simulink model "KillerWhaleModelPneumaticControl"  (R2020b)
settings: Solver=ode15s  StartTime=0.0  StopTime=10  MaxStep=0.01  RelTol=1e-3
model workspace: external: MATLAB File KillerWhaleParams.m (data not in the file)
undefined symbols (not defined in the file or in its folder): frontParams, rearParams, standParams, X, Y, Z
libraries: sm_lib x4301, nesl_utility x6
(part 5 of 66)

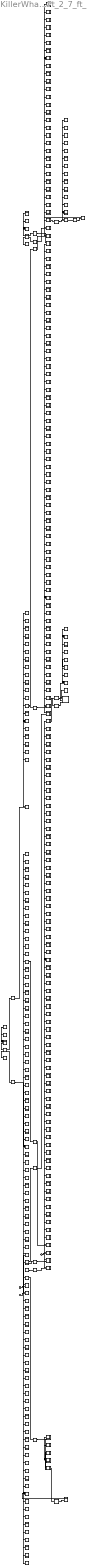
== system KillerWhaleModelPneumaticControl/RearLinkage/Tail_Linkage_Pt_2_7_ft_1 ==
  Bracket_10_RIGID : Subsystem
  Bracket_11_RIGID : Subsystem
  Bracket_12_RIGID : Subsystem
  Bracket_1_RIGID : Subsystem
  Bracket_2_RIGID : Subsystem
  Bracket_3_RIGID : Subsystem
  Bracket_4_RIGID : Subsystem
  Bracket_5_RIGID : Subsystem
  Bracket_6_RIGID : Subsystem
  Bracket_7_RIGID : Subsystem
  Bracket_8_RIGID : Subsystem
  Bracket_9_RIGID : Subsystem
  Cylindrical7 : sm_lib/Joints/Cylindrical Joint  JointMode=Normal  SenseConstraintForce=off  SenseConstraintForceX=off  SenseConstraintForceY=off  SenseConstraintForceZ=off  SenseConstraintTorque=off  SenseConstraintTorqueX=off  SenseConstraintTorqueY=off  SenseConstraintTorqueZ=off  SenseTotalForce=off  SenseTotalForceX=off  SenseTotalForceY=off  SenseTotalForceZ=off  SenseTotalTorque=off  SenseTotalTorqueX=off  SenseTotalTorqueY=off  SenseTotalTorqueZ=off  CompositeWrenchDir=FollowerOnBase  CompositeWrenchFrame=BaseFrame  PzEquilibriumPosition=0  PzEquilibriumPositionUnits=m  PzSpringStiffness=0  PzSpringStiffnessUnits=N/m  PzDampingCoefficient=0  PzDampingCoefficientUnits=N/(m/s)  PzTorqueActuationMode=NoTorque  PzMotionActuationMode=ComputedMotion  PzSensePosition=off  PzSenseVelocity=off  PzSenseAcceleration=off  PzSenseTorqueForce=off  PzSenseLowerLimitTorqueForce=off  PzSenseUpperLimitTorqueForce=off  PzLowerLimitSpecify=off  PzLowerLimitBound=-1  PzLowerLimitBoundUnits=m  PzLowerLimitStiffness=1e6  PzLowerLimitStiffnessUnits=N/m  PzLowerLimitDamping=1e3  PzLowerLimitDampingUnits=N/(m/s)  PzLowerLimitTransitionRegionWidth=1e-4  PzLowerLimitTransitionRegionWidthUnits=m  PzUpperLimitSpecify=off  PzUpperLimitBound=1  PzUpperLimitBoundUnits=m  PzUpperLimitStiffness=1e6  PzUpperLimitStiffnessUnits=N/m  PzUpperLimitDamping=1e3  PzUpperLimitDampingUnits=N/(m/s)  PzUpperLimitTransitionRegionWidth=1e-4  PzUpperLimitTransitionRegionWidthUnits=m  PzPositionTargetSpecify=off  PzPositionTargetPriority=High  PzPositionTargetValue=0  PzPositionTargetValueUnits=m  PzVelocityTargetSpecify=off  PzVelocityTargetPriority=High  PzVelocityTargetValue=0  PzVelocityTargetValueUnits=m/s  RzEquilibriumPosition=0  RzEquilibriumPositionUnits=deg  RzSpringStiffness=0  RzSpringStiffnessUnits=N*m/deg  RzDampingCoefficient=0  RzDampingCoefficientUnits=N*m/(deg/s)  RzTorqueActuationMode=NoTorque  RzMotionActuationMode=ComputedMotion  RzSensePosition=off  RzSenseVelocity=off  RzSenseAcceleration=off  RzSenseTorqueForce=off  RzSenseLowerLimitTorqueForce=off  RzSenseUpperLimitTorqueForce=off  RzLowerLimitSpecify=off  RzLowerLimitBound=-90  RzLowerLimitBoundUnits=deg  RzLowerLimitStiffness=1e4  RzLowerLimitStiffnessUnits=N*m/deg  RzLowerLimitDamping=10  RzLowerLimitDampingUnits=N*m/(deg/s)  RzLowerLimitTransitionRegionWidth=0.1  RzLowerLimitTransitionRegionWidthUnits=deg  RzUpperLimitSpecify=off  RzUpperLimitBound=90  RzUpperLimitBoundUnits=deg  RzUpperLimitStiffness=1e4  RzUpperLimitStiffnessUnits=N*m/deg  RzUpperLimitDamping=10  RzUpperLimitDampingUnits=N*m/(deg/s)  RzUpperLimitTransitionRegionWidth=0.1  RzUpperLimitTransitionRegionWidthUnits=deg  RzPositionTargetSpecify=off  RzPositionTargetPriority=High  RzPositionTargetValue=0  RzPositionTargetValueUnits=deg  RzVelocityTargetSpecify=off  RzVelocityTargetPriority=High  RzVelocityTargetValue=0  RzVelocityTargetValueUnits=deg/s
  Cylindrical8 : sm_lib/Joints/Cylindrical Joint  JointMode=Normal  SenseConstraintForce=off  SenseConstraintForceX=off  SenseConstraintForceY=off  SenseConstraintForceZ=off  SenseConstraintTorque=off  SenseConstraintTorqueX=off  SenseConstraintTorqueY=off  SenseConstraintTorqueZ=off  SenseTotalForce=off  SenseTotalForceX=off  SenseTotalForceY=off  SenseTotalForceZ=off  SenseTotalTorque=off  SenseTotalTorqueX=off  SenseTotalTorqueY=off  SenseTotalTorqueZ=off  CompositeWrenchDir=FollowerOnBase  CompositeWrenchFrame=BaseFrame  PzEquilibriumPosition=0  PzEquilibriumPositionUnits=m  PzSpringStiffness=0  PzSpringStiffnessUnits=N/m  PzDampingCoefficient=0  PzDampingCoefficientUnits=N/(m/s)  PzTorqueActuationMode=NoTorque  PzMotionActuationMode=ComputedMotion  PzSensePosition=off  PzSenseVelocity=off  PzSenseAcceleration=off  PzSenseTorqueForce=off  PzSenseLowerLimitTorqueForce=off  PzSenseUpperLimitTorqueForce=off  PzLowerLimitSpecify=off  PzLowerLimitBound=-1  PzLowerLimitBoundUnits=m  PzLowerLimitStiffness=1e6  PzLowerLimitStiffnessUnits=N/m  PzLowerLimitDamping=1e3  PzLowerLimitDampingUnits=N/(m/s)  PzLowerLimitTransitionRegionWidth=1e-4  PzLowerLimitTransitionRegionWidthUnits=m  PzUpperLimitSpecify=off  PzUpperLimitBound=1  PzUpperLimitBoundUnits=m  PzUpperLimitStiffness=1e6  PzUpperLimitStiffnessUnits=N/m  PzUpperLimitDamping=1e3  PzUpperLimitDampingUnits=N/(m/s)  PzUpperLimitTransitionRegionWidth=1e-4  PzUpperLimitTransitionRegionWidthUnits=m  PzPositionTargetSpecify=off  PzPositionTargetPriority=High  PzPositionTargetValue=0  PzPositionTargetValueUnits=m  PzVelocityTargetSpecify=off  PzVelocityTargetPriority=High  PzVelocityTargetValue=0  PzVelocityTargetValueUnits=m/s  RzEquilibriumPosition=0  RzEquilibriumPositionUnits=deg  RzSpringStiffness=0  RzSpringStiffnessUnits=N*m/deg  RzDampingCoefficient=0  RzDampingCoefficientUnits=N*m/(deg/s)  RzTorqueActuationMode=NoTorque  RzMotionActuationMode=ComputedMotion  RzSensePosition=off  RzSenseVelocity=off  RzSenseAcceleration=off  RzSenseTorqueForce=off  RzSenseLowerLimitTorqueForce=off  RzSenseUpperLimitTorqueForce=off  RzLowerLimitSpecify=off  RzLowerLimitBound=-90  RzLowerLimitBoundUnits=deg  RzLowerLimitStiffness=1e4  RzLowerLimitStiffnessUnits=N*m/deg  RzLowerLimitDamping=10  RzLowerLimitDampingUnits=N*m/(deg/s)  RzLowerLimitTransitionRegionWidth=0.1  RzLowerLimitTransitionRegionWidthUnits=deg  RzUpperLimitSpecify=off  RzUpperLimitBound=90  RzUpperLimitBoundUnits=deg  RzUpperLimitStiffness=1e4  RzUpperLimitStiffnessUnits=N*m/deg  RzUpperLimitDamping=10  RzUpperLimitDampingUnits=N*m/(deg/s)  RzUpperLimitTransitionRegionWidth=0.1  RzUpperLimitTransitionRegionWidthUnits=deg  RzPositionTargetSpecify=off  RzPositionTargetPriority=High  RzPositionTargetValue=0  RzPositionTargetValueUnits=deg  RzVelocityTargetSpecify=off  RzVelocityTargetPriority=High  RzVelocityTargetValue=0  RzVelocityTargetValueUnits=deg/s
  Frame_Part_1_RIGID : Subsystem
  Frame_Part_1_RIGID1 : Subsystem
  Frame_Part_1_RIGID2 : Subsystem
  Frame_Part_1_RIGID3 : Subsystem
  Frame_Part_1_RIGID4 : Subsystem
  Frame_Part_2_RIGID : Subsystem
  Frame_Part_2_RIGID1 : Subsystem
  Frame_Part_2_RIGID2 : Subsystem
  Frame_Part_2_RIGID3 : Subsystem
  Frame_Part_2_RIGID4 : Subsystem
  Frame_Part_3_RIGID : Subsystem
  Frame_Part_4_RIGID : Subsystem
  Hinge_10_RIGID : Subsystem
  Hinge_11_RIGID : Subsystem
  Hinge_12_RIGID : Subsystem
  Hinge_13_RIGID : Subsystem
  Hinge_14_RIGID : Subsystem
  Hinge_15_RIGID : Subsystem
  Hinge_1_RIGID : Subsystem
  Hinge_1_RIGID1 : Subsystem
  Hinge_2_RIGID : Subsystem
  Hinge_3_RIGID : Subsystem
  Hinge_4_RIGID : Subsystem
  Hinge_5_RIGID : Subsystem
  Hinge_6_RIGID : Subsystem
  Hinge_7_RIGID : Subsystem
  Hinge_8_RIGID : Subsystem
  Hinge_9_RIGID : Subsystem
  Lock_tabs_1_RIGID : Subsystem
  Lock_tabs_1_RIGID1 : Subsystem
  Lock_tabs_1_RIGID10 : Subsystem
  Lock_tabs_1_RIGID11 : Subsystem
  Lock_tabs_1_RIGID12 : Subsystem
  Lock_tabs_1_RIGID13 : Subsystem
  Lock_tabs_1_RIGID14 : Subsystem
  Lock_tabs_1_RIGID15 : Subsystem
  Lock_tabs_1_RIGID16 : Subsystem
  Lock_tabs_1_RIGID17 : Subsystem
  Lock_tabs_1_RIGID18 : Subsystem
  Lock_tabs_1_RIGID19 : Subsystem
  Lock_tabs_1_RIGID2 : Subsystem
  Lock_tabs_1_RIGID3 : Subsystem
  Lock_tabs_1_RIGID4 : Subsystem
  Lock_tabs_1_RIGID5 : Subsystem
  Lock_tabs_1_RIGID6 : Subsystem
  Lock_tabs_1_RIGID7 : Subsystem
  Lock_tabs_1_RIGID8 : Subsystem
  Lock_tabs_1_RIGID9 : Subsystem
  ReferenceFrame : sm_lib/Frames and Transforms/Reference Frame
  Revolute1 : sm_lib/Joints/Revolute Joint  JointMode=Normal  SenseConstraintForce=off  SenseConstraintForceX=off  SenseConstraintForceY=off  SenseConstraintForceZ=off  SenseConstraintTorque=off  SenseConstraintTorqueX=off  SenseConstraintTorqueY=off  SenseConstraintTorqueZ=off  SenseTotalForce=off  SenseTotalForceX=off  SenseTotalForceY=off  SenseTotalForceZ=off  SenseTotalTorque=off  SenseTotalTorqueX=off  SenseTotalTorqueY=off  SenseTotalTorqueZ=off  CompositeWrenchDir=FollowerOnBase  CompositeWrenchFrame=BaseFrame  EquilibriumPosition=0  EquilibriumPositionUnits=deg  SpringStiffness=0  SpringStiffnessUnits=N*m/deg  DampingCoefficient=0  DampingCoefficientUnits=N*m/(deg/s)  TorqueActuationMode=NoTorque  MotionActuationMode=ComputedMotion  SensePosition=off  SenseVelocity=off  SenseAcceleration=off  SenseTorqueForce=off  SenseLowerLimitTorqueForce=off  SenseUpperLimitTorqueForce=off  LowerLimitSpecify=off  LowerLimitBound=-90  LowerLimitBoundUnits=deg  LowerLimitStiffness=1e4  LowerLimitStiffnessUnits=N*m/deg  LowerLimitDamping=10  LowerLimitDampingUnits=N*m/(deg/s)  LowerLimitTransitionRegionWidth=0.1  LowerLimitTransitionRegionWidthUnits=deg  UpperLimitSpecify=off  UpperLimitBound=90  UpperLimitBoundUnits=deg  UpperLimitStiffness=1e4  UpperLimitStiffnessUnits=N*m/deg  UpperLimitDamping=10  UpperLimitDampingUnits=N*m/(deg/s)  UpperLimitTransitionRegionWidth=0.1  UpperLimitTransitionRegionWidthUnits=deg  PositionTargetSpecify=on  PositionTargetPriority=Low  PositionTargetValue=rearParams.RevoluteJoint(9).Rz.Pos  PositionTargetValueUnits=deg  VelocityTargetSpecify=off  VelocityTargetPriority=High  VelocityTargetValue=0  VelocityTargetValueUnits=deg/s
  Revolute16 : sm_lib/Joints/Revolute Joint  JointMode=Normal  SenseConstraintForce=off  SenseConstraintForceX=off  SenseConstraintForceY=off  SenseConstraintForceZ=off  SenseConstraintTorque=off  SenseConstraintTorqueX=off  SenseConstraintTorqueY=off  SenseConstraintTorqueZ=off  SenseTotalForce=off  SenseTotalForceX=off  SenseTotalForceY=off  SenseTotalForceZ=off  SenseTotalTorque=off  SenseTotalTorqueX=off  SenseTotalTorqueY=off  SenseTotalTorqueZ=off  CompositeWrenchDir=FollowerOnBase  CompositeWrenchFrame=BaseFrame  EquilibriumPosition=0  EquilibriumPositionUnits=deg  SpringStiffness=0  SpringStiffnessUnits=N*m/deg  DampingCoefficient=0  DampingCoefficientUnits=N*m/(deg/s)  TorqueActuationMode=NoTorque  MotionActuationMode=ComputedMotion  SensePosition=off  SenseVelocity=off  SenseAcceleration=off  SenseTorqueForce=off  SenseLowerLimitTorqueForce=off  SenseUpperLimitTorqueForce=off  LowerLimitSpecify=off  LowerLimitBound=-90  LowerLimitBoundUnits=deg  LowerLimitStiffness=1e4  LowerLimitStiffnessUnits=N*m/deg  LowerLimitDamping=10  LowerLimitDampingUnits=N*m/(deg/s)  LowerLimitTransitionRegionWidth=0.1  LowerLimitTransitionRegionWidthUnits=deg  UpperLimitSpecify=off  UpperLimitBound=90  UpperLimitBoundUnits=deg  UpperLimitStiffness=1e4  UpperLimitStiffnessUnits=N*m/deg  UpperLimitDamping=10  UpperLimitDampingUnits=N*m/(deg/s)  UpperLimitTransitionRegionWidth=0.1  UpperLimitTransitionRegionWidthUnits=deg  PositionTargetSpecify=on  PositionTargetPriority=Low  PositionTargetValue=rearParams.RevoluteJoint(4).Rz.Pos  PositionTargetValueUnits=deg  VelocityTargetSpecify=off  VelocityTargetPriority=High  VelocityTargetValue=0  VelocityTargetValueUnits=deg/s
  Revolute18 : sm_lib/Joints/Revolute Joint  JointMode=Normal  SenseConstraintForce=off  SenseConstraintForceX=off  SenseConstraintForceY=off  SenseConstraintForceZ=off  SenseConstraintTorque=off  SenseConstraintTorqueX=off  SenseConstraintTorqueY=off  SenseConstraintTorqueZ=off  SenseTotalForce=off  SenseTotalForceX=off  SenseTotalForceY=off  SenseTotalForceZ=off  SenseTotalTorque=off  SenseTotalTorqueX=off  SenseTotalTorqueY=off  SenseTotalTorqueZ=off  CompositeWrenchDir=FollowerOnBase  CompositeWrenchFrame=BaseFrame  EquilibriumPosition=0  EquilibriumPositionUnits=deg  SpringStiffness=0  SpringStiffnessUnits=N*m/deg  DampingCoefficient=0  DampingCoefficientUnits=N*m/(deg/s)  TorqueActuationMode=NoTorque  MotionActuationMode=ComputedMotion  SensePosition=off  SenseVelocity=off  SenseAcceleration=off  SenseTorqueForce=off  SenseLowerLimitTorqueForce=off  SenseUpperLimitTorqueForce=off  LowerLimitSpecify=off  LowerLimitBound=-90  LowerLimitBoundUnits=deg  LowerLimitStiffness=1e4  LowerLimitStiffnessUnits=N*m/deg  LowerLimitDamping=10  LowerLimitDampingUnits=N*m/(deg/s)  LowerLimitTransitionRegionWidth=0.1  LowerLimitTransitionRegionWidthUnits=deg  UpperLimitSpecify=off  UpperLimitBound=90  UpperLimitBoundUnits=deg  UpperLimitStiffness=1e4  UpperLimitStiffnessUnits=N*m/deg  UpperLimitDamping=10  UpperLimitDampingUnits=N*m/(deg/s)  UpperLimitTransitionRegionWidth=0.1  UpperLimitTransitionRegionWidthUnits=deg  PositionTargetSpecify=on  PositionTargetPriority=Low  PositionTargetValue=rearParams.RevoluteJoint(10).Rz.Pos  PositionTargetValueUnits=deg  VelocityTargetSpecify=off  VelocityTargetPriority=High  VelocityTargetValue=0  VelocityTargetValueUnits=deg/s
  Revolute2 : sm_lib/Joints/Revolute Joint  JointMode=Normal  SenseConstraintForce=off  SenseConstraintForceX=off  SenseConstraintForceY=off  SenseConstraintForceZ=off  SenseConstraintTorque=off  SenseConstraintTorqueX=off  SenseConstraintTorqueY=off  SenseConstraintTorqueZ=off  SenseTotalForce=off  SenseTotalForceX=off  SenseTotalForceY=off  SenseTotalForceZ=off  SenseTotalTorque=off  SenseTotalTorqueX=off  SenseTotalTorqueY=off  SenseTotalTorqueZ=off  CompositeWrenchDir=FollowerOnBase  CompositeWrenchFrame=BaseFrame  EquilibriumPosition=0  EquilibriumPositionUnits=deg  SpringStiffness=0  SpringStiffnessUnits=N*m/deg  DampingCoefficient=0  DampingCoefficientUnits=N*m/(deg/s)  TorqueActuationMode=NoTorque  MotionActuationMode=ComputedMotion  SensePosition=off  SenseVelocity=off  SenseAcceleration=off  SenseTorqueForce=off  SenseLowerLimitTorqueForce=off  SenseUpperLimitTorqueForce=off  LowerLimitSpecify=off  LowerLimitBound=-90  LowerLimitBoundUnits=deg  LowerLimitStiffness=1e4  LowerLimitStiffnessUnits=N*m/deg  LowerLimitDamping=10  LowerLimitDampingUnits=N*m/(deg/s)  LowerLimitTransitionRegionWidth=0.1  LowerLimitTransitionRegionWidthUnits=deg  UpperLimitSpecify=off  UpperLimitBound=90  UpperLimitBoundUnits=deg  UpperLimitStiffness=1e4  UpperLimitStiffnessUnits=N*m/deg  UpperLimitDamping=10  UpperLimitDampingUnits=N*m/(deg/s)  UpperLimitTransitionRegionWidth=0.1  UpperLimitTransitionRegionWidthUnits=deg  PositionTargetSpecify=on  PositionTargetPriority=Low  PositionTargetValue=rearParams.RevoluteJoint(8).Rz.Pos  PositionTargetValueUnits=deg  VelocityTargetSpecify=off  VelocityTargetPriority=High  VelocityTargetValue=0  VelocityTargetValueUnits=deg/s
  Revolute21 : sm_lib/Joints/Revolute Joint  JointMode=Normal  SenseConstraintForce=off  SenseConstraintForceX=off  SenseConstraintForceY=off  SenseConstraintForceZ=off  SenseConstraintTorque=off  SenseConstraintTorqueX=off  SenseConstraintTorqueY=off  SenseConstraintTorqueZ=off  SenseTotalForce=off  SenseTotalForceX=off  SenseTotalForceY=off  SenseTotalForceZ=off  SenseTotalTorque=off  SenseTotalTorqueX=off  SenseTotalTorqueY=off  SenseTotalTorqueZ=off  CompositeWrenchDir=FollowerOnBase  CompositeWrenchFrame=BaseFrame  EquilibriumPosition=0  EquilibriumPositionUnits=deg  SpringStiffness=0  SpringStiffnessUnits=N*m/deg  DampingCoefficient=0  DampingCoefficientUnits=N*m/(deg/s)  TorqueActuationMode=NoTorque  MotionActuationMode=ComputedMotion  SensePosition=off  SenseVelocity=off  SenseAcceleration=off  SenseTorqueForce=off  SenseLowerLimitTorqueForce=off  SenseUpperLimitTorqueForce=off  LowerLimitSpecify=off  LowerLimitBound=-90  LowerLimitBoundUnits=deg  LowerLimitStiffness=1e4  LowerLimitStiffnessUnits=N*m/deg  LowerLimitDamping=10  LowerLimitDampingUnits=N*m/(deg/s)  LowerLimitTransitionRegionWidth=0.1  LowerLimitTransitionRegionWidthUnits=deg  UpperLimitSpecify=off  UpperLimitBound=90  UpperLimitBoundUnits=deg  UpperLimitStiffness=1e4  UpperLimitStiffnessUnits=N*m/deg  UpperLimitDamping=10  UpperLimitDampingUnits=N*m/(deg/s)  UpperLimitTransitionRegionWidth=0.1  UpperLimitTransitionRegionWidthUnits=deg  PositionTargetSpecify=off  PositionTargetPriority=High  PositionTargetValue=0  PositionTargetValueUnits=deg  VelocityTargetSpecify=off  VelocityTargetPriority=High  VelocityTargetValue=0  VelocityTargetValueUnits=deg/s
  Revolute23 : sm_lib/Joints/Revolute Joint  JointMode=Normal  SenseConstraintForce=off  SenseConstraintForceX=off  SenseConstraintForceY=off  SenseConstraintForceZ=off  SenseConstraintTorque=off  SenseConstraintTorqueX=off  SenseConstraintTorqueY=off  SenseConstraintTorqueZ=off  SenseTotalForce=off  SenseTotalForceX=off  SenseTotalForceY=off  SenseTotalForceZ=off  SenseTotalTorque=off  SenseTotalTorqueX=off  SenseTotalTorqueY=off  SenseTotalTorqueZ=off  CompositeWrenchDir=FollowerOnBase  CompositeWrenchFrame=BaseFrame  EquilibriumPosition=0  EquilibriumPositionUnits=deg  SpringStiffness=0  SpringStiffnessUnits=N*m/deg  DampingCoefficient=0  DampingCoefficientUnits=N*m/(deg/s)  TorqueActuationMode=NoTorque  MotionActuationMode=ComputedMotion  SensePosition=off  SenseVelocity=off  SenseAcceleration=off  SenseTorqueForce=off  SenseLowerLimitTorqueForce=off  SenseUpperLimitTorqueForce=off  LowerLimitSpecify=off  LowerLimitBound=-90  LowerLimitBoundUnits=deg  LowerLimitStiffness=1e4  LowerLimitStiffnessUnits=N*m/deg  LowerLimitDamping=10  LowerLimitDampingUnits=N*m/(deg/s)  LowerLimitTransitionRegionWidth=0.1  LowerLimitTransitionRegionWidthUnits=deg  UpperLimitSpecify=off  UpperLimitBound=90  UpperLimitBoundUnits=deg  UpperLimitStiffness=1e4  UpperLimitStiffnessUnits=N*m/deg  UpperLimitDamping=10  UpperLimitDampingUnits=N*m/(deg/s)  UpperLimitTransitionRegionWidth=0.1  UpperLimitTransitionRegionWidthUnits=deg  PositionTargetSpecify=on  PositionTargetPriority=Low  PositionTargetValue=rearParams.RevoluteJoint(13).Rz.Pos  PositionTargetValueUnits=deg  VelocityTargetSpecify=off  VelocityTargetPriority=High  VelocityTargetValue=0  VelocityTargetValueUnits=deg/s
  Revolute25 : sm_lib/Joints/Revolute Joint  JointMode=Normal  SenseConstraintForce=off  SenseConstraintForceX=off  SenseConstraintForceY=off  SenseConstraintForceZ=off  SenseConstraintTorque=off  SenseConstraintTorqueX=off  SenseConstraintTorqueY=off  SenseConstraintTorqueZ=off  SenseTotalForce=off  SenseTotalForceX=off  SenseTotalForceY=off  SenseTotalForceZ=off  SenseTotalTorque=off  SenseTotalTorqueX=off  SenseTotalTorqueY=off  SenseTotalTorqueZ=off  CompositeWrenchDir=FollowerOnBase  CompositeWrenchFrame=BaseFrame  EquilibriumPosition=0  EquilibriumPositionUnits=deg  SpringStiffness=0  SpringStiffnessUnits=N*m/deg  DampingCoefficient=0  DampingCoefficientUnits=N*m/(deg/s)  TorqueActuationMode=NoTorque  MotionActuationMode=ComputedMotion  SensePosition=off  SenseVelocity=off  SenseAcceleration=off  SenseTorqueForce=off  SenseLowerLimitTorqueForce=off  SenseUpperLimitTorqueForce=off  LowerLimitSpecify=off  LowerLimitBound=-90  LowerLimitBoundUnits=deg  LowerLimitStiffness=1e4  LowerLimitStiffnessUnits=N*m/deg  LowerLimitDamping=10  LowerLimitDampingUnits=N*m/(deg/s)  LowerLimitTransitionRegionWidth=0.1  LowerLimitTransitionRegionWidthUnits=deg  UpperLimitSpecify=off  UpperLimitBound=90  UpperLimitBoundUnits=deg  UpperLimitStiffness=1e4  UpperLimitStiffnessUnits=N*m/deg  UpperLimitDamping=10  UpperLimitDampingUnits=N*m/(deg/s)  UpperLimitTransitionRegionWidth=0.1  UpperLimitTransitionRegionWidthUnits=deg  PositionTargetSpecify=on  PositionTargetPriority=Low  PositionTargetValue=rearParams.RevoluteJoint(5).Rz.Pos  PositionTargetValueUnits=deg  VelocityTargetSpecify=off  VelocityTargetPriority=High  VelocityTargetValue=0  VelocityTargetValueUnits=deg/s
  Revolute26 : sm_lib/Joints/Revolute Joint  JointMode=Normal  SenseConstraintForce=off  SenseConstraintForceX=off  SenseConstraintForceY=off  SenseConstraintForceZ=off  SenseConstraintTorque=off  SenseConstraintTorqueX=off  SenseConstraintTorqueY=off  SenseConstraintTorqueZ=off  SenseTotalForce=off  SenseTotalForceX=off  SenseTotalForceY=off  SenseTotalForceZ=off  SenseTotalTorque=off  SenseTotalTorqueX=off  SenseTotalTorqueY=off  SenseTotalTorqueZ=off  CompositeWrenchDir=FollowerOnBase  CompositeWrenchFrame=BaseFrame  EquilibriumPosition=0  EquilibriumPositionUnits=deg  SpringStiffness=0  SpringStiffnessUnits=N*m/deg  DampingCoefficient=0  DampingCoefficientUnits=N*m/(deg/s)  TorqueActuationMode=NoTorque  MotionActuationMode=ComputedMotion  SensePosition=off  SenseVelocity=off  SenseAcceleration=off  SenseTorqueForce=off  SenseLowerLimitTorqueForce=off  SenseUpperLimitTorqueForce=off  LowerLimitSpecify=off  LowerLimitBound=-90  LowerLimitBoundUnits=deg  LowerLimitStiffness=1e4  LowerLimitStiffnessUnits=N*m/deg  LowerLimitDamping=10  LowerLimitDampingUnits=N*m/(deg/s)  LowerLimitTransitionRegionWidth=0.1  LowerLimitTransitionRegionWidthUnits=deg  UpperLimitSpecify=off  UpperLimitBound=90  UpperLimitBoundUnits=deg  UpperLimitStiffness=1e4  UpperLimitStiffnessUnits=N*m/deg  UpperLimitDamping=10  UpperLimitDampingUnits=N*m/(deg/s)  UpperLimitTransitionRegionWidth=0.1  UpperLimitTransitionRegionWidthUnits=deg  PositionTargetSpecify=off  PositionTargetPriority=High  PositionTargetValue=0  PositionTargetValueUnits=deg  VelocityTargetSpecify=off  VelocityTargetPriority=High  VelocityTargetValue=0  VelocityTargetValueUnits=deg/s
  Revolute3 : sm_lib/Joints/Revolute Joint  JointMode=Normal  SenseConstraintForce=off  SenseConstraintForceX=off  SenseConstraintForceY=off  SenseConstraintForceZ=off  SenseConstraintTorque=off  SenseConstraintTorqueX=off  SenseConstraintTorqueY=off  SenseConstraintTorqueZ=off  SenseTotalForce=off  SenseTotalForceX=off  SenseTotalForceY=off  SenseTotalForceZ=off  SenseTotalTorque=off  SenseTotalTorqueX=off  SenseTotalTorqueY=off  SenseTotalTorqueZ=off  CompositeWrenchDir=FollowerOnBase  CompositeWrenchFrame=BaseFrame  EquilibriumPosition=0  EquilibriumPositionUnits=deg  SpringStiffness=0  SpringStiffnessUnits=N*m/deg  DampingCoefficient=0  DampingCoefficientUnits=N*m/(deg/s)  TorqueActuationMode=NoTorque  MotionActuationMode=ComputedMotion  SensePosition=off  SenseVelocity=off  SenseAcceleration=off  SenseTorqueForce=off  SenseLowerLimitTorqueForce=off  SenseUpperLimitTorqueForce=off  LowerLimitSpecify=off  LowerLimitBound=-90  LowerLimitBoundUnits=deg  LowerLimitStiffness=1e4  LowerLimitStiffnessUnits=N*m/deg  LowerLimitDamping=10  LowerLimitDampingUnits=N*m/(deg/s)  LowerLimitTransitionRegionWidth=0.1  LowerLimitTransitionRegionWidthUnits=deg  UpperLimitSpecify=off  UpperLimitBound=90  UpperLimitBoundUnits=deg  UpperLimitStiffness=1e4  UpperLimitStiffnessUnits=N*m/deg  UpperLimitDamping=10  UpperLimitDampingUnits=N*m/(deg/s)  UpperLimitTransitionRegionWidth=0.1  UpperLimitTransitionRegionWidthUnits=deg  PositionTargetSpecify=on  PositionTargetPriority=Low  PositionTargetValue=rearParams.RevoluteJoint(12).Rz.Pos  PositionTargetValueUnits=deg  VelocityTargetSpecify=off  VelocityTargetPriority=High  VelocityTargetValue=0  VelocityTargetValueUnits=deg/s
  Revolute4 : sm_lib/Joints/Revolute Joint  JointMode=Normal  SenseConstraintForce=off  SenseConstraintForceX=off  SenseConstraintForceY=off  SenseConstraintForceZ=off  SenseConstraintTorque=off  SenseConstraintTorqueX=off  SenseConstraintTorqueY=off  SenseConstraintTorqueZ=off  SenseTotalForce=off  SenseTotalForceX=off  SenseTotalForceY=off  SenseTotalForceZ=off  SenseTotalTorque=off  SenseTotalTorqueX=off  SenseTotalTorqueY=off  SenseTotalTorqueZ=off  CompositeWrenchDir=FollowerOnBase  CompositeWrenchFrame=BaseFrame  EquilibriumPosition=0  EquilibriumPositionUnits=deg  SpringStiffness=0  SpringStiffnessUnits=N*m/deg  DampingCoefficient=0  DampingCoefficientUnits=N*m/(deg/s)  TorqueActuationMode=NoTorque  MotionActuationMode=ComputedMotion  SensePosition=off  SenseVelocity=off  SenseAcceleration=off  SenseTorqueForce=off  SenseLowerLimitTorqueForce=off  SenseUpperLimitTorqueForce=off  LowerLimitSpecify=off  LowerLimitBound=-90  LowerLimitBoundUnits=deg  LowerLimitStiffness=1e4  LowerLimitStiffnessUnits=N*m/deg  LowerLimitDamping=10  LowerLimitDampingUnits=N*m/(deg/s)  LowerLimitTransitionRegionWidth=0.1  LowerLimitTransitionRegionWidthUnits=deg  UpperLimitSpecify=off  UpperLimitBound=90  UpperLimitBoundUnits=deg  UpperLimitStiffness=1e4  UpperLimitStiffnessUnits=N*m/deg  UpperLimitDamping=10  UpperLimitDampingUnits=N*m/(deg/s)  UpperLimitTransitionRegionWidth=0.1  UpperLimitTransitionRegionWidthUnits=deg  PositionTargetSpecify=on  PositionTargetPriority=Low  PositionTargetValue=rearParams.RevoluteJoint(6).Rz.Pos  PositionTargetValueUnits=deg  VelocityTargetSpecify=off  VelocityTargetPriority=High  VelocityTargetValue=0  VelocityTargetValueUnits=deg/s
  Revolute5 : sm_lib/Joints/Revolute Joint  JointMode=Normal  SenseConstraintForce=off  SenseConstraintForceX=off  SenseConstraintForceY=off  SenseConstraintForceZ=off  SenseConstraintTorque=off  SenseConstraintTorqueX=off  SenseConstraintTorqueY=off  SenseConstraintTorqueZ=off  SenseTotalForce=off  SenseTotalForceX=off  SenseTotalForceY=off  SenseTotalForceZ=off  SenseTotalTorque=off  SenseTotalTorqueX=off  SenseTotalTorqueY=off  SenseTotalTorqueZ=off  CompositeWrenchDir=FollowerOnBase  CompositeWrenchFrame=BaseFrame  EquilibriumPosition=0  EquilibriumPositionUnits=deg  SpringStiffness=0  SpringStiffnessUnits=N*m/deg  DampingCoefficient=0  DampingCoefficientUnits=N*m/(deg/s)  TorqueActuationMode=NoTorque  MotionActuationMode=ComputedMotion  SensePosition=off  SenseVelocity=off  SenseAcceleration=off  SenseTorqueForce=off  SenseLowerLimitTorqueForce=off  SenseUpperLimitTorqueForce=off  LowerLimitSpecify=off  LowerLimitBound=-90  LowerLimitBoundUnits=deg  LowerLimitStiffness=1e4  LowerLimitStiffnessUnits=N*m/deg  LowerLimitDamping=10  LowerLimitDampingUnits=N*m/(deg/s)  LowerLimitTransitionRegionWidth=0.1  LowerLimitTransitionRegionWidthUnits=deg  UpperLimitSpecify=off  UpperLimitBound=90  UpperLimitBoundUnits=deg  UpperLimitStiffness=1e4  UpperLimitStiffnessUnits=N*m/deg  UpperLimitDamping=10  UpperLimitDampingUnits=N*m/(deg/s)  UpperLimitTransitionRegionWidth=0.1  UpperLimitTransitionRegionWidthUnits=deg  PositionTargetSpecify=off  PositionTargetPriority=High  PositionTargetValue=0  PositionTargetValueUnits=deg  VelocityTargetSpecify=off  VelocityTargetPriority=High  VelocityTargetValue=0  VelocityTargetValueUnits=deg/s
  Revolute6 : sm_lib/Joints/Revolute Joint  JointMode=Normal  SenseConstraintForce=off  SenseConstraintForceX=off  SenseConstraintForceY=off  SenseConstraintForceZ=off  SenseConstraintTorque=off  SenseConstraintTorqueX=off  SenseConstraintTorqueY=off  SenseConstraintTorqueZ=off  SenseTotalForce=off  SenseTotalForceX=off  SenseTotalForceY=off  SenseTotalForceZ=off  SenseTotalTorque=off  SenseTotalTorqueX=off  SenseTotalTorqueY=off  SenseTotalTorqueZ=off  CompositeWrenchDir=FollowerOnBase  CompositeWrenchFrame=BaseFrame  EquilibriumPosition=0  EquilibriumPositionUnits=deg  SpringStiffness=0  SpringStiffnessUnits=N*m/deg  DampingCoefficient=0  DampingCoefficientUnits=N*m/(deg/s)  TorqueActuationMode=NoTorque  MotionActuationMode=ComputedMotion  SensePosition=off  SenseVelocity=off  SenseAcceleration=off  SenseTorqueForce=off  SenseLowerLimitTorqueForce=off  SenseUpperLimitTorqueForce=off  LowerLimitSpecify=off  LowerLimitBound=-90  LowerLimitBoundUnits=deg  LowerLimitStiffness=1e4  LowerLimitStiffnessUnits=N*m/deg  LowerLimitDamping=10  LowerLimitDampingUnits=N*m/(deg/s)  LowerLimitTransitionRegionWidth=0.1  LowerLimitTransitionRegionWidthUnits=deg  UpperLimitSpecify=off  UpperLimitBound=90  UpperLimitBoundUnits=deg  UpperLimitStiffness=1e4  UpperLimitStiffnessUnits=N*m/deg  UpperLimitDamping=10  UpperLimitDampingUnits=N*m/(deg/s)  UpperLimitTransitionRegionWidth=0.1  UpperLimitTransitionRegionWidthUnits=deg  PositionTargetSpecify=on  PositionTargetPriority=Low  PositionTargetValue=rearParams.RevoluteJoint(2).Rz.Pos  PositionTargetValueUnits=deg  VelocityTargetSpecify=off  VelocityTargetPriority=High  VelocityTargetValue=0  VelocityTargetValueUnits=deg/s
  Revolute7 : sm_lib/Joints/Revolute Joint  JointMode=Normal  SenseConstraintForce=off  SenseConstraintForceX=off  SenseConstraintForceY=off  SenseConstraintForceZ=off  SenseConstraintTorque=off  SenseConstraintTorqueX=off  SenseConstraintTorqueY=off  SenseConstraintTorqueZ=off  SenseTotalForce=off  SenseTotalForceX=off  SenseTotalForceY=off  SenseTotalForceZ=off  SenseTotalTorque=off  SenseTotalTorqueX=off  SenseTotalTorqueY=off  SenseTotalTorqueZ=off  CompositeWrenchDir=FollowerOnBase  CompositeWrenchFrame=BaseFrame  EquilibriumPosition=0  EquilibriumPositionUnits=deg  SpringStiffness=0  SpringStiffnessUnits=N*m/deg  DampingCoefficient=0  DampingCoefficientUnits=N*m/(deg/s)  TorqueActuationMode=NoTorque  MotionActuationMode=ComputedMotion  SensePosition=off  SenseVelocity=off  SenseAcceleration=off  SenseTorqueForce=off  SenseLowerLimitTorqueForce=off  SenseUpperLimitTorqueForce=off  LowerLimitSpecify=off  LowerLimitBound=-90  LowerLimitBoundUnits=deg  LowerLimitStiffness=1e4  LowerLimitStiffnessUnits=N*m/deg  LowerLimitDamping=10  LowerLimitDampingUnits=N*m/(deg/s)  LowerLimitTransitionRegionWidth=0.1  LowerLimitTransitionRegionWidthUnits=deg  UpperLimitSpecify=off  UpperLimitBound=90  UpperLimitBoundUnits=deg  UpperLimitStiffness=1e4  UpperLimitStiffnessUnits=N*m/deg  UpperLimitDamping=10  UpperLimitDampingUnits=N*m/(deg/s)  UpperLimitTransitionRegionWidth=0.1  UpperLimitTransitionRegionWidthUnits=deg  PositionTargetSpecify=on  PositionTargetPriority=Low  PositionTargetValue=rearParams.RevoluteJoint(7).Rz.Pos  PositionTargetValueUnits=deg  VelocityTargetSpecify=off  VelocityTargetPriority=High  VelocityTargetValue=0  VelocityTargetValueUnits=deg/s
  Screw_8_1_2_in_1_RIGID : Subsystem
  Screw_8_1_2_in_1_RIGID1 : Subsystem
  Screw_8_1_2_in_1_RIGID10 : Subsystem
  Screw_8_1_2_in_1_RIGID11 : Subsystem
  Screw_8_1_2_in_1_RIGID12 : Subsystem
  Screw_8_1_2_in_1_RIGID13 : Subsystem
  Screw_8_1_2_in_1_RIGID14 : Subsystem
  Screw_8_1_2_in_1_RIGID15 : Subsystem
  Screw_8_1_2_in_1_RIGID16 : Subsystem
  Screw_8_1_2_in_1_RIGID17 : Subsystem
  Screw_8_1_2_in_1_RIGID18 : Subsystem
  Screw_8_1_2_in_1_RIGID19 : Subsystem
  Screw_8_1_2_in_1_RIGID2 : Subsystem
  Screw_8_1_2_in_1_RIGID20 : Subsystem
  Screw_8_1_2_in_1_RIGID21 : Subsystem
  Screw_8_1_2_in_1_RIGID22 : Subsystem
  Screw_8_1_2_in_1_RIGID23 : Subsystem
  Screw_8_1_2_in_1_RIGID24 : Subsystem
  Screw_8_1_2_in_1_RIGID25 : Subsystem
  Screw_8_1_2_in_1_RIGID26 : Subsystem
  Screw_8_1_2_in_1_RIGID27 : Subsystem
  Screw_8_1_2_in_1_RIGID28 : Subsystem
  Screw_8_1_2_in_1_RIGID29 : Subsystem
  Screw_8_1_2_in_1_RIGID3 : Subsystem
  Screw_8_1_2_in_1_RIGID4 : Subsystem
  Screw_8_1_2_in_1_RIGID5 : Subsystem
  Screw_8_1_2_in_1_RIGID6 : Subsystem
  Screw_8_1_2_in_1_RIGID7 : Subsystem
  Screw_8_1_2_in_1_RIGID8 : Subsystem
  Screw_8_1_2_in_1_RIGID9 : Subsystem
  Screw_8_3_4_in_1_RIGID : Subsystem
  Screw_8_3_4_in_1_RIGID1 : Subsystem
  Screw_8_3_4_in_1_RIGID2 : Subsystem
  Screw_8_3_4_in_1_RIGID3 : Subsystem
  Set_Screw_4_1_4_in_10_RIGID : Subsystem
  Set_Screw_4_1_4_in_11_RIGID : Subsystem
  Set_Screw_4_1_4_in_12_RIGID : Subsystem
  Set_Screw_4_1_4_in_1_RIGID : Subsystem
  Set_Screw_4_1_4_in_2_RIGID : Subsystem
  Set_Screw_4_1_4_in_3_RIGID : Subsystem
  Set_Screw_4_1_4_in_4_RIGID : Subsystem
  Set_Screw_4_1_4_in_5_RIGID : Subsystem
  Set_Screw_4_1_4_in_6_RIGID : Subsystem
  Set_Screw_4_1_4_in_7_RIGID : Subsystem
  Set_Screw_4_1_4_in_8_RIGID : Subsystem
  Set_Screw_4_1_4_in_9_RIGID : Subsystem
  Sleeve_1_RIGID : Subsystem
  Sleeve_1_RIGID1 : Subsystem
  Sleeve_1_RIGID2 : Subsystem
  Sleeve_1_RIGID3 : Subsystem
  Sleeve_1_RIGID4 : Subsystem
  Sleeve_1_RIGID5 : Subsystem
  Sleeve_1_RIGID6 : Subsystem
  Sleeve_1_RIGID7 : Subsystem
  Sleeve_1_RIGID8 : Subsystem
  Spacer_1_RIGID : Subsystem
  Spacer_1_RIGID1 : Subsystem
  Spacer_1_RIGID10 : Subsystem
  Spacer_1_RIGID11 : Subsystem
  Spacer_1_RIGID12 : Subsystem
  Spacer_1_RIGID13 : Subsystem
  Spacer_1_RIGID14 : Subsystem
  Spacer_1_RIGID15 : Subsystem
  Spacer_1_RIGID16 : Subsystem
  Spacer_1_RIGID17 : Subsystem
  Spacer_1_RIGID18 : Subsystem
  Spacer_1_RIGID19 : Subsystem
  Spacer_1_RIGID2 : Subsystem
  Spacer_1_RIGID20 : Subsystem
  Spacer_1_RIGID21 : Subsystem
  Spacer_1_RIGID22 : Subsystem
  Spacer_1_RIGID23 : Subsystem
  Spacer_1_RIGID24 : Subsystem
  Spacer_1_RIGID25 : Subsystem
  Spacer_1_RIGID26 : Subsystem
  Spacer_1_RIGID27 : Subsystem
  Spacer_1_RIGID28 : Subsystem
  Spacer_1_RIGID29 : Subsystem
  Spacer_1_RIGID3 : Subsystem
  Spacer_1_RIGID30 : Subsystem
  Spacer_1_RIGID31 : Subsystem
  Spacer_1_RIGID32 : Subsystem
  Spacer_1_RIGID33 : Subsystem
  Spacer_1_RIGID4 : Subsystem
  Spacer_1_RIGID5 : Subsystem
  Spacer_1_RIGID6 : Subsystem
  Spacer_1_RIGID7 : Subsystem
  Spacer_1_RIGID8 : Subsystem
  Spacer_1_RIGID9 : Subsystem
  Spring_Pin_1_8_in_OD_1_4_in_L_10_RIGID : Subsystem
  Spring_Pin_1_8_in_OD_1_4_in_L_10_RIGID1 : Subsystem
  Spring_Pin_1_8_in_OD_1_4_in_L_10_RIGID2 : Subsystem
  Spring_Pin_1_8_in_OD_1_4_in_L_11_RIGID : Subsystem
  Spring_Pin_1_8_in_OD_1_4_in_L_11_RIGID1 : Subsystem
  Spring_Pin_1_8_in_OD_1_4_in_L_11_RIGID2 : Subsystem
  Spring_Pin_1_8_in_OD_1_4_in_L_12_RIGID : Subsystem
  Spring_Pin_1_8_in_OD_1_4_in_L_12_RIGID1 : Subsystem
  Spring_Pin_1_8_in_OD_1_4_in_L_12_RIGID2 : Subsystem
  Spring_Pin_1_8_in_OD_1_4_in_L_13_RIGID : Subsystem
  Spring_Pin_1_8_in_OD_1_4_in_L_13_RIGID1 : Subsystem
  Spring_Pin_1_8_in_OD_1_4_in_L_13_RIGID2 : Subsystem
  Spring_Pin_1_8_in_OD_1_4_in_L_14_RIGID : Subsystem
  Spring_Pin_1_8_in_OD_1_4_in_L_14_RIGID1 : Subsystem
  Spring_Pin_1_8_in_OD_1_4_in_L_14_RIGID2 : Subsystem
  Spring_Pin_1_8_in_OD_1_4_in_L_15_RIGID : Subsystem
  Spring_Pin_1_8_in_OD_1_4_in_L_15_RIGID1 : Subsystem
  Spring_Pin_1_8_in_OD_1_4_in_L_15_RIGID2 : Subsystem
  Spring_Pin_1_8_in_OD_1_4_in_L_16_RIGID : Subsystem
  Spring_Pin_1_8_in_OD_1_4_in_L_16_RIGID1 : Subsystem
  Spring_Pin_1_8_in_OD_1_4_in_L_16_RIGID2 : Subsystem
  Spring_Pin_1_8_in_OD_1_4_in_L_17_RIGID : Subsystem
  Spring_Pin_1_8_in_OD_1_4_in_L_17_RIGID1 : Subsystem
  Spring_Pin_1_8_in_OD_1_4_in_L_17_RIGID2 : Subsystem
  Spring_Pin_1_8_in_OD_1_4_in_L_18_RIGID : Subsystem
  Spring_Pin_1_8_in_OD_1_4_in_L_18_RIGID1 : Subsystem
  Spring_Pin_1_8_in_OD_1_4_in_L_18_RIGID2 : Subsystem
  Spring_Pin_1_8_in_OD_1_4_in_L_19_RIGID : Subsystem
  Spring_Pin_1_8_in_OD_1_4_in_L_19_RIGID1 : Subsystem
  Spring_Pin_1_8_in_OD_1_4_in_L_19_RIGID2 : Subsystem
  Spring_Pin_1_8_in_OD_1_4_in_L_1_RIGID : Subsystem
  Spring_Pin_1_8_in_OD_1_4_in_L_1_RIGID1 : Subsystem
  Spring_Pin_1_8_in_OD_1_4_in_L_1_RIGID2 : Subsystem
  Spring_Pin_1_8_in_OD_1_4_in_L_20_RIGID : Subsystem
  Spring_Pin_1_8_in_OD_1_4_in_L_20_RIGID1 : Subsystem
  Spring_Pin_1_8_in_OD_1_4_in_L_20_RIGID2 : Subsystem
  Spring_Pin_1_8_in_OD_1_4_in_L_21_RIGID : Subsystem
  Spring_Pin_1_8_in_OD_1_4_in_L_21_RIGID1 : Subsystem
  Spring_Pin_1_8_in_OD_1_4_in_L_21_RIGID2 : Subsystem
  Spring_Pin_1_8_in_OD_1_4_in_L_22_RIGID : Subsystem
  Spring_Pin_1_8_in_OD_1_4_in_L_22_RIGID1 : Subsystem
  Spring_Pin_1_8_in_OD_1_4_in_L_22_RIGID2 : Subsystem
  Spring_Pin_1_8_in_OD_1_4_in_L_23_RIGID : Subsystem
  Spring_Pin_1_8_in_OD_1_4_in_L_23_RIGID1 : Subsystem
  Spring_Pin_1_8_in_OD_1_4_in_L_23_RIGID2 : Subsystem
  Spring_Pin_1_8_in_OD_1_4_in_L_24_RIGID : Subsystem
  Spring_Pin_1_8_in_OD_1_4_in_L_24_RIGID1 : Subsystem
  Spring_Pin_1_8_in_OD_1_4_in_L_24_RIGID2 : Subsystem
  Spring_Pin_1_8_in_OD_1_4_in_L_25_RIGID : Subsystem
  Spring_Pin_1_8_in_OD_1_4_in_L_25_RIGID1 : Subsystem
  Spring_Pin_1_8_in_OD_1_4_in_L_25_RIGID2 : Subsystem
  Spring_Pin_1_8_in_OD_1_4_in_L_26_RIGID : Subsystem
  Spring_Pin_1_8_in_OD_1_4_in_L_26_RIGID1 : Subsystem
  Spring_Pin_1_8_in_OD_1_4_in_L_26_RIGID2 : Subsystem
  Spring_Pin_1_8_in_OD_1_4_in_L_27_RIGID : Subsystem
  Spring_Pin_1_8_in_OD_1_4_in_L_27_RIGID1 : Subsystem
  Spring_Pin_1_8_in_OD_1_4_in_L_27_RIGID2 : Subsystem
  Spring_Pin_1_8_in_OD_1_4_in_L_28_RIGID : Subsystem
  Spring_Pin_1_8_in_OD_1_4_in_L_28_RIGID1 : Subsystem
  Spring_Pin_1_8_in_OD_1_4_in_L_28_RIGID2 : Subsystem
  Spring_Pin_1_8_in_OD_1_4_in_L_29_RIGID : Subsystem
  Spring_Pin_1_8_in_OD_1_4_in_L_29_RIGID1 : Subsystem
  Spring_Pin_1_8_in_OD_1_4_in_L_29_RIGID2 : Subsystem
  Spring_Pin_1_8_in_OD_1_4_in_L_2_RIGID : Subsystem
  Spring_Pin_1_8_in_OD_1_4_in_L_2_RIGID1 : Subsystem
  Spring_Pin_1_8_in_OD_1_4_in_L_2_RIGID2 : Subsystem
  Spring_Pin_1_8_in_OD_1_4_in_L_30_RIGID : Subsystem
  Spring_Pin_1_8_in_OD_1_4_in_L_30_RIGID1 : Subsystem
  Spring_Pin_1_8_in_OD_1_4_in_L_30_RIGID2 : Subsystem
  Spring_Pin_1_8_in_OD_1_4_in_L_3_RIGID : Subsystem
  Spring_Pin_1_8_in_OD_1_4_in_L_3_RIGID1 : Subsystem
  Spring_Pin_1_8_in_OD_1_4_in_L_3_RIGID2 : Subsystem
  Spring_Pin_1_8_in_OD_1_4_in_L_4_RIGID : Subsystem
  Spring_Pin_1_8_in_OD_1_4_in_L_4_RIGID1 : Subsystem
  Spring_Pin_1_8_in_OD_1_4_in_L_4_RIGID2 : Subsystem
  Spring_Pin_1_8_in_OD_1_4_in_L_5_RIGID : Subsystem
  Spring_Pin_1_8_in_OD_1_4_in_L_5_RIGID1 : Subsystem
  Spring_Pin_1_8_in_OD_1_4_in_L_5_RIGID2 : Subsystem
  Spring_Pin_1_8_in_OD_1_4_in_L_6_RIGID : Subsystem
  Spring_Pin_1_8_in_OD_1_4_in_L_6_RIGID1 : Subsystem
  Spring_Pin_1_8_in_OD_1_4_in_L_6_RIGID2 : Subsystem
  Spring_Pin_1_8_in_OD_1_4_in_L_7_RIGID : Subsystem
  Spring_Pin_1_8_in_OD_1_4_in_L_7_RIGID1 : Subsystem
  Spring_Pin_1_8_in_OD_1_4_in_L_7_RIGID2 : Subsystem
  Spring_Pin_1_8_in_OD_1_4_in_L_8_RIGID : Subsystem
  Spring_Pin_1_8_in_OD_1_4_in_L_8_RIGID1 : Subsystem
  Spring_Pin_1_8_in_OD_1_4_in_L_8_RIGID2 : Subsystem
  Spring_Pin_1_8_in_OD_1_4_in_L_9_RIGID : Subsystem
  Spring_Pin_1_8_in_OD_1_4_in_L_9_RIGID1 : Subsystem
  Spring_Pin_1_8_in_OD_1_4_in_L_9_RIGID2 : Subsystem
  Spring_Pin_3_32_in_OD_3_16_in_L_1_RIGID : Subsystem
  Spring_Pin_3_32_in_OD_3_16_in_L_1_RIGID1 : Subsystem
  Spring_Pin_3_32_in_OD_3_16_in_L_1_RIGID2 : Subsystem
  Spring_Pin_3_32_in_OD_3_16_in_L_1_RIGID3 : Subsystem
  Spring_Pin_3_32_in_OD_3_16_in_L_1_RIGID4 : Subsystem
  Spring_Pin_3_32_in_OD_3_16_in_L_1_RIGID5 : Subsystem
  Standoff_1_RIGID : Subsystem
  Transform : sm_lib/Frames and Transforms/Rigid Transform  TranslationMethod=Cartesian  TranslationStandardOffset=0  TranslationLengthUnit=in  TranslationStandardAxis=+Z  TranslationCartesianOffset=rearParams.RigidTransform(789).translation  TranslationROffset=0  TranslationROffsetUnits=m  TranslationZOffset=0  TranslationZOffsetUnits=m  TranslationThetaOffset=0  TranslationThetaOffsetUnits=deg  RotationMethod=ArbitraryAxis  RotationAngleUnits=rad  RotationStandardAxis=+Z  RotationAngle=rearParams.RigidTransform(789).angle  RotationArbitraryAxis=rearParams.RigidTransform(789).axis  FollAlignAxisA=+X  BaseAlignAxisA=+Y  FollAlignAxisB=+Y  BaseAlignAxisB=+Z  RotationSequenceAxes=FollowerAxes  RotationSequence=XYX  RotationSequenceAngles=[0 0 0]  RotationSequenceAnglesUnits=deg  RotationMatrix=[1 0 0; 0 1 0; 0 0 1]
  Washer_8_1_RIGID : Subsystem
  Washer_8_1_RIGID1 : Subsystem
  Washer_8_1_RIGID10 : Subsystem
  Washer_8_1_RIGID11 : Subsystem
  Washer_8_1_RIGID12 : Subsystem
  Washer_8_1_RIGID13 : Subsystem
  Washer_8_1_RIGID14 : Subsystem
  Washer_8_1_RIGID15 : Subsystem
  Washer_8_1_RIGID16 : Subsystem
  Washer_8_1_RIGID17 : Subsystem
  Washer_8_1_RIGID18 : Subsystem
  Washer_8_1_RIGID19 : Subsystem
  Washer_8_1_RIGID2 : Subsystem
  Washer_8_1_RIGID20 : Subsystem
  Washer_8_1_RIGID21 : Subsystem
  Washer_8_1_RIGID22 : Subsystem
  Washer_8_1_RIGID23 : Subsystem
  Washer_8_1_RIGID24 : Subsystem
  Washer_8_1_RIGID25 : Subsystem
  Washer_8_1_RIGID26 : Subsystem
  Washer_8_1_RIGID27 : Subsystem
  Washer_8_1_RIGID28 : Subsystem
  Washer_8_1_RIGID29 : Subsystem
  Washer_8_1_RIGID3 : Subsystem
  Washer_8_1_RIGID30 : Subsystem
  Washer_8_1_RIGID31 : Subsystem
  Washer_8_1_RIGID32 : Subsystem
  Washer_8_1_RIGID33 : Subsystem
  Washer_8_1_RIGID4 : Subsystem
  Washer_8_1_RIGID5 : Subsystem
  Washer_8_1_RIGID6 : Subsystem
  Washer_8_1_RIGID7 : Subsystem
  Washer_8_1_RIGID8 : Subsystem
  Washer_8_1_RIGID9 : Subsystem
  braces1_1_RIGID : Subsystem
  braces1_2_RIGID : Subsystem
  braces1_3_RIGID : Subsystem
  braces2_1_RIGID : Subsystem
  braces2_2_RIGID : Subsystem
  braces2_3_RIGID : Subsystem
  braces3_1_RIGID : Subsystem
  braces3_2_RIGID : Subsystem
  braces3_3_RIGID : Subsystem
  braces4_1_RIGID : Subsystem
  braces4_2_RIGID : Subsystem
  braces4_3_RIGID : Subsystem
  bulkheads1_1_RIGID : Subsystem
  bulkheads1_2_RIGID : Subsystem
  bulkheads1_3_RIGID : Subsystem
  bulkheads1_4_RIGID : Subsystem
  bulkheads1_5_RIGID : Subsystem
  link6l_1_RIGID : Subsystem
  link6r_1_RIGID : Subsystem
  link7l_1_RIGID : Subsystem
  link7r_1_RIGID : Subsystem
  link8l_1_RIGID : Subsystem
  link8r_1_RIGID : Subsystem
  link9l_1_RIGID : Subsystem
  link9r_1_RIGID : Subsystem
  tail11_1_RIGID : Subsystem
  tail12_1_RIGID : Subsystem
  tail13_1_RIGID : Subsystem
  tail15_1_RIGID : Subsystem
  tail1_1_RIGID : Subsystem
  tail2_1_RIGID : Subsystem
  tail3_1_RIGID : Subsystem
  tail4_1_RIGID : Subsystem
  tail5_1_RIGID : Subsystem
  tail6_1_RIGID : Subsystem
  tail7_1_RIGID : Subsystem
  tail8_1_RIGID : Subsystem
  tail9_1_RIGID : Subsystem
  tail_14_1_RIGID : Subsystem
  F2 : PMIOPort  Side=Left
  F1 : PMIOPort  Port=2  Side=Left
  F : PMIOPort  Port=3  Side=Left
  connections:
  Bracket_11_RIGID/LConn1 -- Bracket_10_RIGID/LConn1 -- Frame_Part_1_RIGID4/LConn1 -- Frame_Part_2_RIGID3/LConn1 -- Hinge_1_RIGID/LConn1 -- Lock_tabs_1_RIGID/LConn1 -- Lock_tabs_1_RIGID3/LConn1 -- Screw_8_1_2_in_1_RIGID1/LConn1 -- Screw_8_1_2_in_1_RIGID6/LConn1 -- Set_Screw_4_1_4_in_4_RIGID/LConn1 -- Set_Screw_4_1_4_in_6_RIGID/LConn1 -- Spacer_1_RIGID20/LConn1 -- Spacer_1_RIGID9/LConn1 -- Spring_Pin_1_8_in_OD_1_4_in_L_12_RIGID1/LConn1 -- Spring_Pin_1_8_in_OD_1_4_in_L_13_RIGID/LConn1 -- Spring_Pin_1_8_in_OD_1_4_in_L_15_RIGID/LConn1 -- Spring_Pin_1_8_in_OD_1_4_in_L_19_RIGID/LConn1 -- Spring_Pin_1_8_in_OD_1_4_in_L_21_RIGID2/LConn1 -- Spring_Pin_1_8_in_OD_1_4_in_L_23_RIGID/LConn1 -- Washer_8_1_RIGID2/LConn1 -- Washer_8_1_RIGID21/LConn1
  braces3_2_RIGID/LConn1 -- braces3_1_RIGID/LConn2 -- braces3_3_RIGID/LConn1
  link9l_1_RIGID/LConn2 -- link9r_1_RIGID/LConn1
  Frame_Part_2_RIGID2/LConn1 -- Frame_Part_1_RIGID3/LConn1 -- Frame_Part_3_RIGID/LConn1 -- Frame_Part_4_RIGID/LConn1 -- Hinge_1_RIGID1/LConn1 -- Hinge_3_RIGID/LConn1 -- Hinge_8_RIGID/LConn1 -- Hinge_9_RIGID/LConn1 -- Lock_tabs_1_RIGID1/LConn1 -- Lock_tabs_1_RIGID18/LConn1 -- Lock_tabs_1_RIGID2/LConn1 -- Lock_tabs_1_RIGID5/LConn1 -- Lock_tabs_1_RIGID6/LConn1 -- Lock_tabs_1_RIGID9/LConn1 -- Screw_8_1_2_in_1_RIGID/LConn1 -- Screw_8_1_2_in_1_RIGID12/LConn1 -- Screw_8_1_2_in_1_RIGID14/LConn1 -- Screw_8_1_2_in_1_RIGID18/LConn1 -- Screw_8_1_2_in_1_RIGID21/LConn1 -- Screw_8_1_2_in_1_RIGID24/LConn1 -- Screw_8_3_4_in_1_RIGID/LConn1 -- Screw_8_3_4_in_1_RIGID1/LConn1 -- Screw_8_3_4_in_1_RIGID2/LConn1 -- Screw_8_3_4_in_1_RIGID3/LConn1 -- Sleeve_1_RIGID/LConn1 -- Sleeve_1_RIGID2/LConn1 -- Sleeve_1_RIGID3/LConn1 -- Spacer_1_RIGID1/LConn1 -- Spacer_1_RIGID14/LConn1 -- Spacer_1_RIGID16/LConn1 -- Spacer_1_RIGID18/LConn1 -- Spacer_1_RIGID19/LConn1 -- Spacer_1_RIGID21/LConn1 -- Spacer_1_RIGID24/LConn1 -- Spacer_1_RIGID25/LConn1 -- Spacer_1_RIGID30/LConn1 -- Spacer_1_RIGID7/LConn1 -- Spring_Pin_1_8_in_OD_1_4_in_L_13_RIGID2/LConn1 -- Spring_Pin_1_8_in_OD_1_4_in_L_14_RIGID2/LConn1 -- Spring_Pin_1_8_in_OD_1_4_in_L_15_RIGID1/LConn1 -- Spring_Pin_1_8_in_OD_1_4_in_L_18_RIGID/LConn1 -- Spring_Pin_1_8_in_OD_1_4_in_L_18_RIGID1/LConn1 -- Spring_Pin_1_8_in_OD_1_4_in_L_21_RIGID/LConn1 -- Spring_Pin_1_8_in_OD_1_4_in_L_22_RIGID/LConn1 -- Spring_Pin_1_8_in_OD_1_4_in_L_23_RIGID2/LConn1 -- Spring_Pin_1_8_in_OD_1_4_in_L_25_RIGID2/LConn1 -- Spring_Pin_1_8_in_OD_1_4_in_L_26_RIGID2/LConn1 -- Spring_Pin_1_8_in_OD_1_4_in_L_27_RIGID1/LConn1 -- Spring_Pin_1_8_in_OD_1_4_in_L_28_RIGID/LConn1 -- Spring_Pin_1_8_in_OD_1_4_in_L_29_RIGID2/LConn1 -- Spring_Pin_1_8_in_OD_1_4_in_L_3_RIGID2/LConn1 -- Spring_Pin_1_8_in_OD_1_4_in_L_6_RIGID/LConn1 -- Spring_Pin_1_8_in_OD_1_4_in_L_6_RIGID2/LConn1 -- Spring_Pin_1_8_in_OD_1_4_in_L_9_RIGID1/LConn1 -- Spring_Pin_1_8_in_OD_1_4_in_L_9_RIGID2/LConn1 -- Spring_Pin_3_32_in_OD_3_16_in_L_1_RIGID/LConn1 -- Spring_Pin_3_32_in_OD_3_16_in_L_1_RIGID1/LConn1 -- Spring_Pin_3_32_in_OD_3_16_in_L_1_RIGID2/LConn1 -- Spring_Pin_3_32_in_OD_3_16_in_L_1_RIGID3/LConn1 -- Spring_Pin_3_32_in_OD_3_16_in_L_1_RIGID4/LConn1 -- Spring_Pin_3_32_in_OD_3_16_in_L_1_RIGID5/LConn1 -- Standoff_1_RIGID/LConn1 -- Washer_8_1_RIGID14/LConn1 -- Washer_8_1_RIGID15/LConn1 -- Washer_8_1_RIGID16/LConn1 -- Washer_8_1_RIGID17/LConn1 -- Washer_8_1_RIGID20/LConn1 -- Washer_8_1_RIGID30/LConn1 -- Washer_8_1_RIGID33/LConn1 -- Washer_8_1_RIGID6/LConn1 -- Washer_8_1_RIGID7/LConn1 -- Washer_8_1_RIGID9/LConn1
  Frame_Part_2_RIGID/LConn1 -- Frame_Part_1_RIGID1/LConn1 -- Hinge_11_RIGID/LConn1 -- Hinge_14_RIGID/LConn1 -- Hinge_15_RIGID/LConn1 -- Hinge_2_RIGID/LConn1 -- Lock_tabs_1_RIGID10/LConn1 -- Lock_tabs_1_RIGID16/LConn1 -- Lock_tabs_1_RIGID17/LConn1 -- Lock_tabs_1_RIGID19/LConn1 -- Screw_8_1_2_in_1_RIGID10/LConn1 -- Screw_8_1_2_in_1_RIGID17/LConn1 -- Screw_8_1_2_in_1_RIGID19/LConn1 -- Screw_8_1_2_in_1_RIGID2/LConn1 -- Screw_8_1_2_in_1_RIGID23/LConn1 -- Screw_8_1_2_in_1_RIGID26/LConn1 -- Screw_8_1_2_in_1_RIGID28/LConn1 -- Screw_8_1_2_in_1_RIGID7/LConn1 -- Sleeve_1_RIGID4/LConn1 -- Sleeve_1_RIGID5/LConn1 -- Sleeve_1_RIGID6/LConn1 -- Sleeve_1_RIGID7/LConn1 -- Spacer_1_RIGID23/LConn2 -- Spacer_1_RIGID28/LConn1 -- Spacer_1_RIGID31/LConn1 -- Spacer_1_RIGID32/LConn1 -- Spacer_1_RIGID33/LConn1 -- Spacer_1_RIGID5/LConn1 -- Spacer_1_RIGID6/LConn1 -- Spacer_1_RIGID8/LConn1 -- Spring_Pin_1_8_in_OD_1_4_in_L_10_RIGID/LConn1 -- Spring_Pin_1_8_in_OD_1_4_in_L_12_RIGID2/LConn1 -- Spring_Pin_1_8_in_OD_1_4_in_L_15_RIGID2/LConn1 -- Spring_Pin_1_8_in_OD_1_4_in_L_17_RIGID1/LConn1 -- Spring_Pin_1_8_in_OD_1_4_in_L_17_RIGID2/LConn1 -- Spring_Pin_1_8_in_OD_1_4_in_L_19_RIGID2/LConn1 -- Spring_Pin_1_8_in_OD_1_4_in_L_20_RIGID1/LConn1 -- Spring_Pin_1_8_in_OD_1_4_in_L_20_RIGID2/LConn1 -- Spring_Pin_1_8_in_OD_1_4_in_L_22_RIGID1/LConn1 -- Spring_Pin_1_8_in_OD_1_4_in_L_24_RIGID/LConn1 -- Spring_Pin_1_8_in_OD_1_4_in_L_24_RIGID1/LConn1 -- Spring_Pin_1_8_in_OD_1_4_in_L_24_RIGID2/LConn1 -- Spring_Pin_1_8_in_OD_1_4_in_L_25_RIGID1/LConn1 -- Spring_Pin_1_8_in_OD_1_4_in_L_28_RIGID1/LConn1 -- Spring_Pin_1_8_in_OD_1_4_in_L_29_RIGID/LConn1 -- Spring_Pin_1_8_in_OD_1_4_in_L_29_RIGID1/LConn1 -- Spring_Pin_1_8_in_OD_1_4_in_L_2_RIGID/LConn1 -- Spring_Pin_1_8_in_OD_1_4_in_L_30_RIGID/LConn1 -- Spring_Pin_1_8_in_OD_1_4_in_L_30_RIGID1/LConn1 -- Spring_Pin_1_8_in_OD_1_4_in_L_30_RIGID2/LConn1 -- Spring_Pin_1_8_in_OD_1_4_in_L_4_RIGID/LConn1 -- Spring_Pin_1_8_in_OD_1_4_in_L_4_RIGID1/LConn1 -- Spring_Pin_1_8_in_OD_1_4_in_L_5_RIGID/LConn1 -- Spring_Pin_1_8_in_OD_1_4_in_L_7_RIGID1/LConn1 -- Washer_8_1_RIGID/LConn1 -- Washer_8_1_RIGID12/LConn1 -- Washer_8_1_RIGID13/LConn1 -- Washer_8_1_RIGID19/LConn1 -- Washer_8_1_RIGID22/LConn1 -- Washer_8_1_RIGID23/LConn1 -- Washer_8_1_RIGID28/LConn1 -- Washer_8_1_RIGID29/LConn1
  link8l_1_RIGID/LConn2 -- link8r_1_RIGID/LConn1
  braces4_2_RIGID/LConn1 -- braces4_1_RIGID/LConn1 -- braces4_3_RIGID/LConn1
  link6l_1_RIGID/LConn2 -- link6r_1_RIGID/LConn1
  Frame_Part_2_RIGID4/RConn1 -- Revolute21/LConn1
  Lock_tabs_1_RIGID16/LConn2 -- Revolute21/RConn1
  Cylindrical8/LConn1 -- Frame_Part_2_RIGID4/RConn2
  Cylindrical8/RConn1 -- Lock_tabs_1_RIGID6/LConn2
  Bracket_4_RIGID/LConn1 -- Bracket_1_RIGID/LConn1 -- Bracket_5_RIGID/LConn1 -- Bracket_9_RIGID/LConn1 -- Frame_Part_1_RIGID/LConn1 -- Frame_Part_2_RIGID4/LConn1 -- Hinge_10_RIGID/LConn1 -- Hinge_12_RIGID/LConn1 -- Lock_tabs_1_RIGID12/LConn1 -- Lock_tabs_1_RIGID13/LConn1 -- Screw_8_1_2_in_1_RIGID11/LConn1 -- Screw_8_1_2_in_1_RIGID16/LConn1 -- Screw_8_1_2_in_1_RIGID20/LConn1 -- Screw_8_1_2_in_1_RIGID25/LConn1 -- Set_Screw_4_1_4_in_12_RIGID/LConn1 -- Set_Screw_4_1_4_in_2_RIGID/LConn1 -- Set_Screw_4_1_4_in_3_RIGID/LConn1 -- Set_Screw_4_1_4_in_9_RIGID/LConn1 -- Spacer_1_RIGID/LConn2 -- Spacer_1_RIGID15/LConn1 -- Spacer_1_RIGID2/LConn1 -- Spacer_1_RIGID29/LConn1 -- Spring_Pin_1_8_in_OD_1_4_in_L_11_RIGID1/LConn1 -- Spring_Pin_1_8_in_OD_1_4_in_L_11_RIGID2/LConn1 -- Spring_Pin_1_8_in_OD_1_4_in_L_12_RIGID/LConn1 -- Spring_Pin_1_8_in_OD_1_4_in_L_16_RIGID2/LConn1 -- Spring_Pin_1_8_in_OD_1_4_in_L_17_RIGID/LConn1 -- Spring_Pin_1_8_in_OD_1_4_in_L_23_RIGID1/LConn1 -- Spring_Pin_1_8_in_OD_1_4_in_L_28_RIGID2/LConn1 -- Spring_Pin_1_8_in_OD_1_4_in_L_3_RIGID/LConn1 -- Spring_Pin_1_8_in_OD_1_4_in_L_3_RIGID1/LConn1 -- Spring_Pin_1_8_in_OD_1_4_in_L_6_RIGID1/LConn1 -- Spring_Pin_1_8_in_OD_1_4_in_L_8_RIGID/LConn1 -- Spring_Pin_1_8_in_OD_1_4_in_L_8_RIGID1/LConn1 -- Washer_8_1_RIGID10/LConn1 -- Washer_8_1_RIGID18/LConn1 -- Washer_8_1_RIGID32/LConn1 -- Washer_8_1_RIGID5/LConn1
  Revolute6/LConn1 -- tail6_1_RIGID/RConn1
  Revolute6/RConn1 -- Spacer_1_RIGID12/LConn2
  Revolute5/LConn1 -- Sleeve_1_RIGID1/RConn1
  Revolute5/RConn1 -- tail6_1_RIGID/LConn2
  braces3_1_RIGID/LConn1 -- bulkheads1_2_RIGID/LConn2
  Cylindrical7/LConn1 -- Frame_Part_1_RIGID4/RConn2
  Cylindrical7/RConn1 -- Lock_tabs_1_RIGID17/LConn2
  Frame_Part_2_RIGID1/RConn1 -- Revolute16/LConn1
  Lock_tabs_1_RIGID1/LConn2 -- Revolute16/RConn1
  Revolute25/LConn1 -- link9l_1_RIGID/RConn2
  Bracket_2_RIGID/LConn1 -- Bracket_12_RIGID/LConn1 -- Bracket_3_RIGID/LConn1 -- Bracket_6_RIGID/LConn1 -- Bracket_7_RIGID/LConn1 -- Bracket_8_RIGID/LConn1 -- Frame_Part_1_RIGID2/LConn1 -- Frame_Part_2_RIGID1/LConn1 -- Hinge_4_RIGID/LConn1 -- Hinge_5_RIGID/LConn1 -- Hinge_6_RIGID/LConn1 -- Lock_tabs_1_RIGID14/LConn1 -- Lock_tabs_1_RIGID4/LConn1 -- Screw_8_1_2_in_1_RIGID13/LConn1 -- Screw_8_1_2_in_1_RIGID15/LConn1 -- Screw_8_1_2_in_1_RIGID22/LConn1 -- Screw_8_1_2_in_1_RIGID27/LConn1 -- Screw_8_1_2_in_1_RIGID8/LConn1 -- Screw_8_1_2_in_1_RIGID9/LConn1 -- Set_Screw_4_1_4_in_10_RIGID/LConn1 -- Set_Screw_4_1_4_in_11_RIGID/LConn1 -- Set_Screw_4_1_4_in_1_RIGID/LConn1 -- Set_Screw_4_1_4_in_5_RIGID/LConn1 -- Set_Screw_4_1_4_in_7_RIGID/LConn1 -- Set_Screw_4_1_4_in_8_RIGID/LConn1 -- Spacer_1_RIGID10/LConn1 -- Spacer_1_RIGID13/LConn1 -- Spacer_1_RIGID22/LConn1 -- Spacer_1_RIGID26/LConn1 -- Spacer_1_RIGID3/LConn1 -- Spacer_1_RIGID4/LConn1 -- Spring_Pin_1_8_in_OD_1_4_in_L_11_RIGID/LConn1 -- Spring_Pin_1_8_in_OD_1_4_in_L_13_RIGID1/LConn1 -- Spring_Pin_1_8_in_OD_1_4_in_L_16_RIGID/LConn1 -- Spring_Pin_1_8_in_OD_1_4_in_L_16_RIGID1/LConn1 -- Spring_Pin_1_8_in_OD_1_4_in_L_18_RIGID2/LConn1 -- Spring_Pin_1_8_in_OD_1_4_in_L_19_RIGID1/LConn1 -- Spring_Pin_1_8_in_OD_1_4_in_L_1_RIGID/LConn1 -- Spring_Pin_1_8_in_OD_1_4_in_L_20_RIGID/LConn1 -- Spring_Pin_1_8_in_OD_1_4_in_L_21_RIGID1/LConn1 -- Spring_Pin_1_8_in_OD_1_4_in_L_26_RIGID1/LConn1 -- Spring_Pin_1_8_in_OD_1_4_in_L_27_RIGID/LConn1 -- Spring_Pin_1_8_in_OD_1_4_in_L_2_RIGID1/LConn1 -- Spring_Pin_1_8_in_OD_1_4_in_L_2_RIGID2/LConn1 -- Spring_Pin_1_8_in_OD_1_4_in_L_4_RIGID2/LConn1 -- Spring_Pin_1_8_in_OD_1_4_in_L_5_RIGID1/LConn1 -- Spring_Pin_1_8_in_OD_1_4_in_L_7_RIGID/LConn1 -- Spring_Pin_1_8_in_OD_1_4_in_L_8_RIGID2/LConn1 -- Spring_Pin_1_8_in_OD_1_4_in_L_9_RIGID/LConn1 -- Washer_8_1_RIGID1/LConn1 -- Washer_8_1_RIGID24/LConn1 -- Washer_8_1_RIGID26/LConn1 -- Washer_8_1_RIGID27/LConn1 -- Washer_8_1_RIGID31/LConn1 -- Washer_8_1_RIGID8/LConn1
  Lock_tabs_1_RIGID7/LConn2 -- Revolute25/RConn1
  Revolute4/LConn1 -- link9l_1_RIGID/RConn1
  Revolute4/RConn1 -- Spacer_1_RIGID23/LConn1
  braces2_1_RIGID/LConn2 -- link8l_1_RIGID/LConn1
  Revolute7/LConn1 -- Spacer_1_RIGID32/RConn1
  Revolute7/RConn1 -- link7l_1_RIGID/LConn4
  Revolute2/LConn1 -- Spacer_1_RIGID18/RConn1
  Revolute2/RConn1 -- link7l_1_RIGID/LConn3
  braces3_1_RIGID/LConn3 -- link7l_1_RIGID/LConn1
  braces4_1_RIGID/LConn2 -- link6l_1_RIGID/LConn3
  tail12_1_RIGID/LConn1 -- tail11_1_RIGID/LConn1 -- tail13_1_RIGID/LConn1 -- tail15_1_RIGID/LConn1 -- tail1_1_RIGID/LConn1 -- tail2_1_RIGID/LConn1 -- tail3_1_RIGID/LConn1 -- tail4_1_RIGID/LConn1 -- tail5_1_RIGID/LConn1 -- tail6_1_RIGID/LConn1 -- tail7_1_RIGID/LConn1 -- tail8_1_RIGID/LConn1 -- tail9_1_RIGID/LConn1 -- tail_14_1_RIGID/LConn1
  Revolute1/LConn1 -- Spacer_1_RIGID22/RConn1
  Revolute1/RConn1 -- link6l_1_RIGID/LConn1
  Revolute18/LConn1 -- link6l_1_RIGID/RConn1
  Lock_tabs_1_RIGID12/LConn2 -- Revolute18/RConn1
  Frame_Part_1_RIGID4/RConn1 -- Revolute26/LConn1
  Lock_tabs_1_RIGID8/LConn2 -- Revolute26/RConn1
  Revolute3/LConn1 -- link8l_1_RIGID/RConn2
  Revolute3/RConn1 -- Spacer_1_RIGID/LConn1
  Revolute23/LConn1 -- link8l_1_RIGID/RConn1
  Lock_tabs_1_RIGID/LConn2 -- Revolute23/RConn1
  Hinge_7_RIGID/LConn1 -- Hinge_13_RIGID/LConn1 -- Lock_tabs_1_RIGID11/LConn1 -- Lock_tabs_1_RIGID15/LConn1 -- Lock_tabs_1_RIGID7/LConn1 -- Lock_tabs_1_RIGID8/LConn1 -- Screw_8_1_2_in_1_RIGID29/LConn1 -- Screw_8_1_2_in_1_RIGID3/LConn1 -- Screw_8_1_2_in_1_RIGID4/LConn1 -- Screw_8_1_2_in_1_RIGID5/LConn1 -- Sleeve_1_RIGID1/LConn1 -- Sleeve_1_RIGID8/LConn1 -- Spacer_1_RIGID11/LConn1 -- Spacer_1_RIGID12/LConn1 -- Spacer_1_RIGID17/LConn1 -- Spacer_1_RIGID27/LConn1 -- Spring_Pin_1_8_in_OD_1_4_in_L_10_RIGID1/LConn1 -- Spring_Pin_1_8_in_OD_1_4_in_L_10_RIGID2/LConn1 -- Spring_Pin_1_8_in_OD_1_4_in_L_14_RIGID/LConn1 -- Spring_Pin_1_8_in_OD_1_4_in_L_14_RIGID1/LConn1 -- Spring_Pin_1_8_in_OD_1_4_in_L_1_RIGID1/LConn1 -- Spring_Pin_1_8_in_OD_1_4_in_L_1_RIGID2/LConn1 -- Spring_Pin_1_8_in_OD_1_4_in_L_22_RIGID2/LConn1 -- Spring_Pin_1_8_in_OD_1_4_in_L_25_RIGID/LConn1 -- Spring_Pin_1_8_in_OD_1_4_in_L_26_RIGID/LConn1 -- Spring_Pin_1_8_in_OD_1_4_in_L_27_RIGID2/LConn1 -- Spring_Pin_1_8_in_OD_1_4_in_L_5_RIGID2/LConn1 -- Spring_Pin_1_8_in_OD_1_4_in_L_7_RIGID2/LConn1 -- Washer_8_1_RIGID11/LConn1 -- Washer_8_1_RIGID25/LConn1 -- Washer_8_1_RIGID3/LConn1 -- Washer_8_1_RIGID4/LConn1
  braces1_1_RIGID/LConn2 -- link9l_1_RIGID/LConn1
  Hinge_1_RIGID1/LConn2 -- F/RConn1
  Spacer_1_RIGID13/LConn2 -- F1/RConn1
  Lock_tabs_1_RIGID4/LConn2 -- F2/RConn1
  Frame_Part_3_RIGID/LConn2 -- Transform/RConn1
  ReferenceFrame/RConn1 -- Transform/LConn1
  braces1_2_RIGID/LConn1 -- braces1_1_RIGID/LConn1 -- braces1_3_RIGID/LConn1
  bulkheads1_2_RIGID/LConn1 -- bulkheads1_1_RIGID/LConn1 -- bulkheads1_3_RIGID/LConn1 -- bulkheads1_4_RIGID/LConn1 -- bulkheads1_5_RIGID/LConn1
  braces2_2_RIGID/LConn1 -- braces2_1_RIGID/LConn1 -- braces2_3_RIGID/LConn1
  link7l_1_RIGID/LConn2 -- link7r_1_RIGID/LConn1
